simulink library "Linkage_Arms"  (R2025a)
settings: Solver=VariableStepAuto  StartTime=0.0  StopTime=10.0  RelTol=1e-3
undefined symbols (not defined in the file): Ac, Af, Ar, bcr_mass, clr_bcr, clr_conn_la, clr_conn_pullrod, clr_conn_rod, clr_la, clr_laf, clr_lar, clr_pullrod, clr_rod, clr_ua, hp_arb, hp_bcr_pivot, hp_bcr_shock_heave, hp_bcr_shock_roll, hp_in_f_la, hp_in_f_ua, hp_in_r_la, hp_in_r_ua, hp_la_arb, hp_out_f_la, hp_out_la, hp_out_r_la, hp_out_ua, hp_pullrod_in, hp_pullrod_out, hp_pushrod_in, hp_spr_bcr, hp_spr_bot, hp_uar_rod, hp_upr_rod, la_mass, laf_mass, lar_mass, opc_bcr, opc_conn_la, opc_conn_pullrod, opc_conn_rod, opc_la, opc_laf, opc_lar, opc_pullrod, opc_rod, opc_ua, pullrod_mass, radius_bcr, radius_la, radius_laf, radius_lar, radius_pullrod, radius_rod, radius_ua, rod_mass, size_conn_la, size_conn_pullrod, size_conn_rod, ua_mass ... (+3)
libraries: Suspension_Utilities x29, sm_lib x25
(part 2 of 2)

== system Linkage_Arms/Track Rod ==
  Rod : Suspension_Utilities/Cylinder Between Two Points  hp_b=hp_in.*[1 rhs_rod 1]  hp_f=hp_out.*[1 rhs_rod 1]  Mass=rod_mass  clr_solid=clr_rod  opc_solid=opc_rod  rad_solid=radius_rod
  Vis Rack Rod : sm_lib/Body Elements/Spherical Solid  SphereRadius=size_conn_rod  SphereRadiusUnits=m  ExportEntireGeometry=off  InertiaType=CalculateFromGeometry  BasedOnType=Density  Density=0  DensityUnits=kg/m^3  Mass=1  MassUnits=kg  CenterOfMass=[0 0 0]  CenterOfMassUnits=m  MomentsOfInertia=[1 1 1]  MomentsOfInertiaUnits=kg*m^2  ProductsOfInertia=[0 0 0]  ProductsOfInertiaUnits=kg*m^2  GraphicType=FromGeometry  MarkerShape=Sphere  MarkerSize=10  GraphicVisPropType=SimpleVisualProperties  GraphicDiffuseColor=clr_conn_rod  GraphicOpacity=opc_conn_rod  GraphicSpecularColor=[0.5 0.5 0.5 1.0]  GraphicAmbientColor=[0.15 0.15 0.15 1.0]  GraphicEmissiveColor=[0.0 0.0 0.0 1.0]  GraphicShininess=75  DoExposeReferenceFrame=on  SerializedFrames=<Frames/>
  Vis Upright Steer : sm_lib/Body Elements/Spherical Solid  SphereRadius=size_conn_rod  SphereRadiusUnits=m  ExportEntireGeometry=off  InertiaType=CalculateFromGeometry  BasedOnType=Density  Density=0  DensityUnits=kg/m^3  Mass=1  MassUnits=kg  CenterOfMass=[0 0 0]  CenterOfMassUnits=m  MomentsOfInertia=[1 1 1]  MomentsOfInertiaUnits=kg*m^2  ProductsOfInertia=[0 0 0]  ProductsOfInertiaUnits=kg*m^2  GraphicType=FromGeometry  MarkerShape=Sphere  MarkerSize=10  GraphicVisPropType=SimpleVisualProperties  GraphicDiffuseColor=clr_conn_rod  GraphicOpacity=opc_conn_rod  GraphicSpecularColor=[0.5 0.5 0.5 1.0]  GraphicAmbientColor=[0.15 0.15 0.15 1.0]  GraphicEmissiveColor=[0.0 0.0 0.0 1.0]  GraphicShininess=75  DoExposeReferenceFrame=on  SerializedFrames=<Frames/>
  Rack : PMIOPort  Side=Right
  Upr : PMIOPort  Port=2  Side=Left
  connections:
  Vis Upright Steer/RConn1 -- Rod/RConn1 -- Upr/RConn1
  Rod/LConn1 -- Rack/RConn1 -- Vis Rack Rod/RConn1
